simulink library "csc_sim_mtv_simulation_lib"  (R2014b)
settings: Solver=ode45  StartTime=0.0  StopTime=10.0  RelTol=1e-3
undefined symbols (not defined in the file or in its folder): ini_epoch_seconds, sim_time_step_size, swm_num_switches
libraries: util_common_lib x4, util_info_lib x1, telem_conversion_lib x1, csc_egt_egc_thruster_lib x1, csc_enf_environmental_forces_mtv_lib x1, csc_prs_pressure_system_sim_lib x1, csc_pwr_power_system_sim_lib x1, csc_rigid_body_dynamics_lib x1, csc_sensors_mtv_lib x1, csc_thl_thrusters_mtv_lib x1, csc_thm_thermal_system_sim_lib x1, csu_afm_aerodynamics_lib x1
settings Model: Creator=nkulkarni  LastModifiedBy=Mark Wells

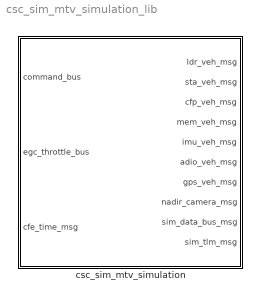
== system csc_sim_mtv_simulation_lib ==
  csc_sim_mtv_simulation : Subsystem  Tag=GSSE; MDL_TICK=THR_SIM_MSG  TreatAsAtomicUnit=on  SystemSampleTime=sim_time_step_size

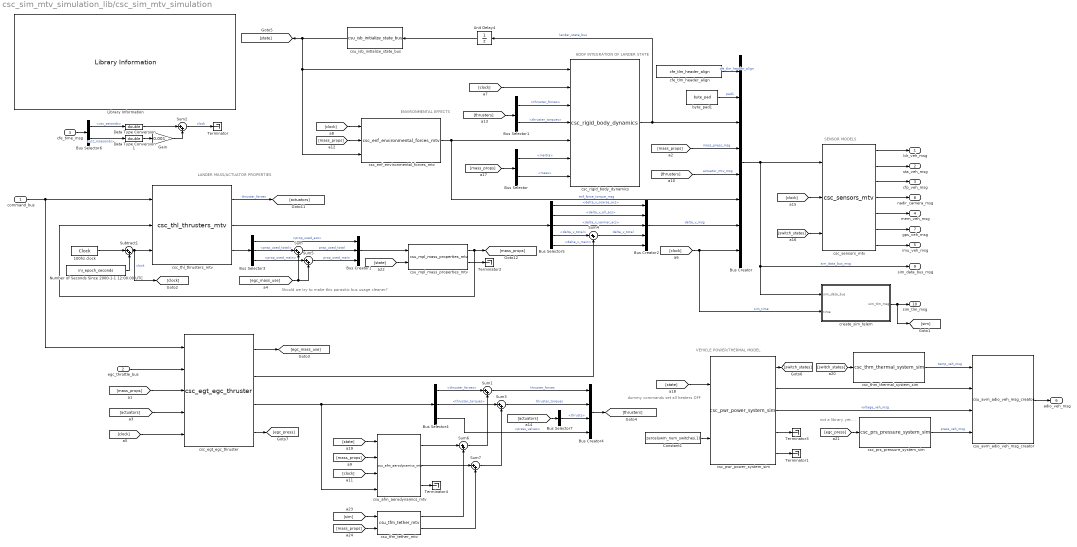
== system csc_sim_mtv_simulation_lib/csc_sim_mtv_simulation ==
  note: Should we try to make this parasitic bus usage cleaner?
  note: SENSOR MODELS
  note: ENVIRONMENTAL EFFECTS
  note: 6DOF INTEGRATION OF LANDER STATE
  note: LANDER MASS/ACTUATOR PROPERTIES
  note: dummy commands set all heaters OFF
  note: VEHICLE POWER/THERMAL MODEL
  note: not a library yet....
  command_bus : Inport
  egc_throttle_bus : Inport  Port=2
  cfe_time_msg : Inport  Port=3  OutDataTypeStr=Bus: cfe_time_msg
  100hz clock : DigitalClock  SampleTime=sim_time_step_size
  Bus Creator : BusCreator  Inputs=8  OutDataTypeStr=Bus: sim_data_mtv_msg  NonVirtualBus=on
  Bus Creator1 : BusCreator  Inputs=3
  Bus Creator2 : BusCreator  Inputs=5
  Bus Creator4 : BusCreator  OutDataTypeStr=Bus: actuator_mtv_msg_t
  Bus Selector : BusSelector  OutputSignals=inertia,mass
  Bus Selector1 : BusSelector  OutputSignals=thruster_forces,thruster_torques
  Bus Selector3 : BusSelector  OutputSignals=prop_used_acs,prop_used_total,prop_used_main
  Bus Selector4 : BusSelector  OutputSignals=thruster_forces,thruster_torques,press_valves
  Bus Selector5 : BusSelector  OutputSignals=delta_v_coarse_acs,delta_v_all_acs,delta_v_vernier_acs,delta_v_total,delta_v_main
  Bus Selector6 : BusSelector  OutputSignals=utc_seconds,utc_mseconds
  Bus Selector7 : BusSelector  OutputSignals=thrusts
  Constant1 : Constant  Value=zeros(swm_num_switches,1)  OutDataTypeStr=double
  Data Type Conversion : DataTypeConversion  OutDataTypeStr=double
  Data Type Conversion1 : DataTypeConversion  OutDataTypeStr=double
  Gain : Gain  Gain=0.001
  Library Information : util_info_lib/Library Information  owner='NONE'
  Number of Seconds Since 2000-1-1 12:00:00 UTC : Constant  Description=|  Value=ini_epoch_seconds
      | Number of Seconds                   
      | July 4, 2014 22:40:00 UTC           
      | Calculate on Web Site:              
      | www.mbari.org/staff/rich/utccalc.htm
  Subtract1 : Sum  Inputs=|++
  Sum{,1..7} (8 alike) : Sum  Inputs=|++
  Terminator{,1..4} (5 alike) : Terminator
  Unit Delay4 : UnitDelay  SampleTime=-1
  byte_pad1 : util_common_lib/byte_pad  n_bytes=4
  cfe_tlm_header_align : util_common_lib/cfe_tlm_header_align
  create_sim_telem : Subsystem
  csc_egt_egc_thruster : csc_egt_egc_thruster_lib/csc_egt_egc_thruster
  csc_enf_environmental_forces_mtv : csc_enf_environmental_forces_mtv_lib/csc_enf_environmental_forces_mtv
  csc_prs_pressure_system_sim : csc_prs_pressure_system_sim_lib/csc_prs_pressure_system_sim
  csc_pwr_power_system_sim : csc_pwr_power_system_sim_lib/csc_pwr_power_system_sim
  csc_rigid_body_dynamics : csc_rigid_body_dynamics_lib/csc_rigid_body_dynamics
  csc_sensors_mtv : csc_sensors_mtv_lib/csc_sensors_mtv
  csc_thl_thrusters_mtv : csc_thl_thrusters_mtv_lib/csc_thl_thrusters_mtv
  csc_thm_thermal_system_sim : csc_thm_thermal_system_sim_lib/csc_thm_thermal_system_sim
  csu_afm_aerodynamics_mtv : csu_afm_aerodynamics_lib/csu_afm_aerodynamics_mtv  SystemSampleTime=-1
  csu_avm_adio_veh_msg_creator : csu_avm_adio_veh_msg_creator_lib/csu_avm_adio_veh_msg_creator
  csu_isb_initialize_state_bus : csu_isb_initialize_state_bus_lib/csu_isb_initialize_state_bus
  csu_mpl_mass_properties_mtv : csu_mpl_mass_properties_mtv_lib/csu_mpl_mass_properties_mtv
  csu_tfm_tether_mtv : csu_tfm_tether_mtv/csu_tfm_tether_mtv
  ldr_veh_msg : Outport
  sta_veh_msg : Outport  Port=2
  cfp_veh_msg : Outport  Port=3
  mem_veh_msg : Outport  Port=4
  imu_veh_msg : Outport  Port=5
  adio_veh_msg : Outport  Port=6
  gps_veh_msg : Outport  Port=7
  nadir_camera_msg : Outport  Port=8
  sim_data_bus_msg : Outport  Port=9
  sim_tlm_msg : Outport  Port=10
  wires:
  Sum7/1 -> Sum3/2
  Sum6/1 -> Sum1/2
  csu_tfm_tether_mtv/2 -> Sum7/2
  csu_afm_aerodynamics_mtv/2 -> Sum7/1
  csu_tfm_tether_mtv/1 -> Sum6/2
  csu_afm_aerodynamics_mtv/1 -> Sum6/1
  [sim] -> csu_tfm_tether_mtv/1
  [mass_props] -> csu_tfm_tether_mtv/2
  Bus Selector4/2 -> Sum3/1  "<thruster_torques>"
  Bus Selector4/1 -> Sum1/1  "<thruster_forces>"
  [state] -> csu_afm_aerodynamics_mtv/1
  [mass_props] -> csu_afm_aerodynamics_mtv/2
  csc_sensors_mtv/7 -> imu_veh_msg/1
  [state] -> csu_mpl_mass_properties_mtv/2
  csc_sensors_mtv/6 -> gps_veh_msg/1
  csu_mpl_mass_properties_mtv/2 -> Terminator2/1
  Bus Selector4/3 -> Bus Creator4/4  "<press_valves>"
  Sum5/1 -> Bus Creator1/3  "prop_used_main"
  [clock] -> csc_egt_egc_thruster/5
  command_bus/1 -> csc_thl_thrusters_mtv/1, csc_egt_egc_thruster/1
  csc_egt_egc_thruster/4 -> [egc_press]
  csc_prs_pressure_system_sim/1 -> csu_avm_adio_veh_msg_creator/4  "press_veh_msg"
  [egc_press] -> csc_prs_pressure_system_sim/1
  csc_pwr_power_system_sim/3 -> csu_avm_adio_veh_msg_creator/3  "voltage_veh_msg"
  csc_pwr_power_system_sim/2 -> csu_avm_adio_veh_msg_creator/2
  csc_thm_thermal_system_sim/1 -> csu_avm_adio_veh_msg_creator/1  "temp_veh_msg"
  csu_avm_adio_veh_msg_creator/1 -> adio_veh_msg/1
  [switch_states] -> csc_thm_thermal_system_sim/1
  Sum2/1 -> Terminator/1  "clock"
  100hz clock/1 -> Subtract1/1
  Number of Seconds Since 2000-1-1 12:00:00 UTC/1 -> Subtract1/2
  csc_sensors_mtv/5 -> mem_veh_msg/1
  [mass_props] -> csc_enf_environmental_forces_mtv/2
  [clock] -> csc_enf_environmental_forces_mtv/1
  csc_thl_thrusters_mtv/1 -> [actuators]  "thruster_forces"
  csc_enf_environmental_forces_mtv/1 -> Bus Creator/6, csc_rigid_body_dynamics/5  "enf_force_torque_msg"
  Bus Selector1/2 -> csc_rigid_body_dynamics/4  "<thruster_torques>"
  Bus Selector1/1 -> csc_rigid_body_dynamics/3  "<thruster_forces>"
  csu_mpl_mass_properties_mtv/1 -> [mass_props], csc_thl_thrusters_mtv/2
  Bus Selector/1 -> csc_rigid_body_dynamics/6  "<inertia>"
  Bus Selector/2 -> csc_rigid_body_dynamics/7  "<mass>"
  [mass_props] -> Bus Creator/4  "mass_props_msg"
  [thrusters] -> Bus Creator/5  "actuator_mtv_msg"
  [thrusters] -> Bus Selector1/1
  [mass_props] -> Bus Selector/1
  csc_rigid_body_dynamics/1 -> Bus Creator/3, Unit Delay4/1  "lander_state_bus"
  Bus Creator/1 -> csc_sensors_mtv/1, sim_data_bus_msg/1, create_sim_telem/1(sim_data_bus)  "sim_data_bus_msg"
  create_sim_telem/1(sim_tlm_msg) -> sim_tlm_msg/1, [sim]
  [clock] -> create_sim_telem/2(time), Bus Creator/8  "sim_time"
  Subtract1/1 -> csc_thl_thrusters_mtv/3, [clock]  "clock"
  byte_pad1/1 -> Bus Creator/2  "pad1"
  csc_thl_thrusters_mtv/3 -> Bus Selector3/1
  csc_egt_egc_thruster/1 -> [egc_mass_use]
  Bus Selector3/2 -> Sum/1  "<prop_used_total>"
  [egc_mass_use] -> Sum/2, Sum5/2
  Sum/1 -> Bus Creator1/2  "prop_used_total"
  Bus Selector3/1 -> Bus Creator1/1  "<prop_used_acs>"
  Bus Selector3/3 -> Sum5/1  "<prop_used_main>"
  Bus Creator1/1 -> csu_mpl_mass_properties_mtv/1
  csc_egt_egc_thruster/2 -> Sum4/2
  Bus Creator2/1 -> Bus Creator/7  "delta_v_msg"
  csc_thl_thrusters_mtv/2 -> Bus Selector5/1
  Bus Selector5/4 -> Sum4/1  "<delta_v_total>"
  Sum4/1 -> Bus Creator2/4  "delta_v_total"
  Bus Selector5/5 -> Bus Creator2/5  "<delta_v_main>"
  Bus Selector5/3 -> Bus Creator2/3  "<delta_v_vernier_acs>"
  Bus Selector5/2 -> Bus Creator2/2  "<delta_v_all_acs>"
  Bus Selector5/1 -> Bus Creator2/1  "<delta_v_coarse_acs>"
  [actuators] -> csc_egt_egc_thruster/4
  [mass_props] -> csc_egt_egc_thruster/3
  egc_throttle_bus/1 -> csc_egt_egc_thruster/2
  cfe_time_msg/1 -> Bus Selector6/1
  Bus Selector6/2 -> Data Type Conversion1/1  "<utc_mseconds>"
  Data Type Conversion/1 -> Sum2/1
  Data Type Conversion1/1 -> Gain/1
  Gain/1 -> Sum2/2
  Bus Selector6/1 -> Data Type Conversion/1  "<utc_seconds>"
  csc_sensors_mtv/1 -> ldr_veh_msg/1
  csc_sensors_mtv/2 -> sta_veh_msg/1
  csc_sensors_mtv/3 -> cfp_veh_msg/1
  csc_sensors_mtv/4 -> nadir_camera_msg/1
  cfe_tlm_header_align/1 -> Bus Creator/1  "cfe_tlm_header_align"
  [clock] -> csc_rigid_body_dynamics/2
  csu_isb_initialize_state_bus/1 -> [state], csc_rigid_body_dynamics/1, csc_enf_environmental_forces_mtv/3
  Unit Delay4/1 -> csu_isb_initialize_state_bus/1
  [clock] -> csc_sensors_mtv/2
  Constant1/1 -> csc_pwr_power_system_sim/2
  [state] -> csc_pwr_power_system_sim/1
  csc_pwr_power_system_sim/1 -> [switch_states]
  csc_pwr_power_system_sim/4 -> Terminator3/1
  csc_pwr_power_system_sim/5 -> Terminator1/1
  [switch_states] -> csc_sensors_mtv/3
  csc_egt_egc_thruster/3 -> csu_afm_aerodynamics_mtv/4, Bus Selector4/1
  Sum1/1 -> Bus Creator4/1  "thruster_forces"
  Bus Creator4/1 -> [thrusters]
  [actuators] -> Bus Selector7/1
  Bus Selector7/1 -> Bus Creator4/3  "<thrusts>"
  Sum3/1 -> Bus Creator4/2  "thruster_torques"
  [clock] -> csu_afm_aerodynamics_mtv/3
  csu_afm_aerodynamics_mtv/3 -> Terminator4/1

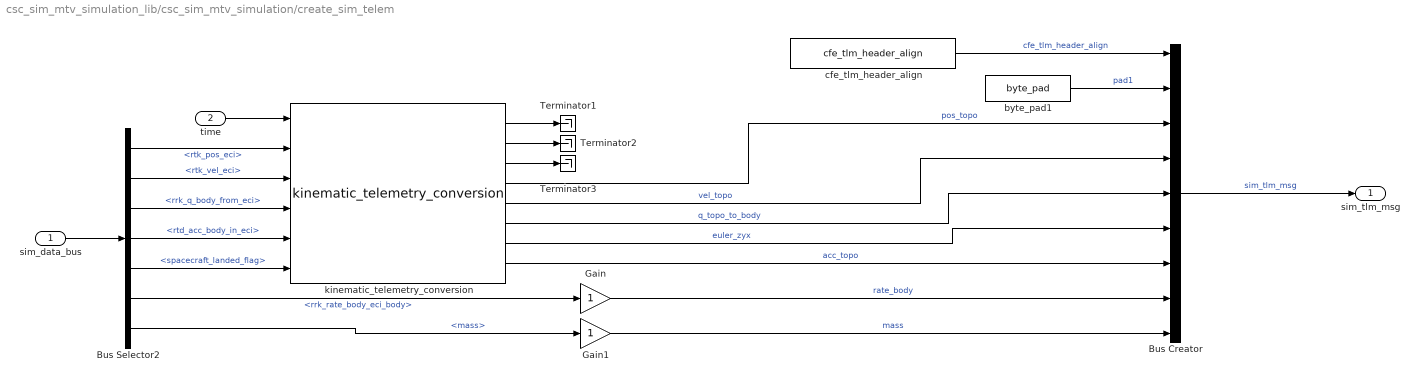
== system csc_sim_mtv_simulation_lib/csc_sim_mtv_simulation/create_sim_telem ==
  sim_data_bus : Inport
  time : Inport  Port=2
  Bus Creator : BusCreator  Inputs=9  OutDataTypeStr=Bus: sim_tlm_msg  NonVirtualBus=on
  Bus Selector2 : BusSelector  OutputSignals=lander_state_bus.rtk_pos_eci,lander_state_bus.rtk_vel_eci,lander_state_bus.rrk_q_body_from_eci,lander_state_bus.rtd_acc_body_in_eci,lander_state_bus.spacecraft_landed_flag,lander_state_bus.rrk_rate_body_eci_body,mass_props_msg.mass
  Gain : Gain
  Gain1 : Gain
  Terminator1 : Terminator
  Terminator2 : Terminator
  Terminator3 : Terminator
  byte_pad1 : util_common_lib/byte_pad  n_bytes=4
  cfe_tlm_header_align : util_common_lib/cfe_tlm_header_align
  kinematic_telemetry_conversion : telem_conversion_lib/kinematic_telemetry_conversion
  sim_tlm_msg : Outport
  wires:
  Bus Selector2/5 -> kinematic_telemetry_conversion/6  "<spacecraft_landed_flag>"
  kinematic_telemetry_conversion/4 -> Bus Creator/3  "pos_topo"
  Gain1/1 -> Bus Creator/9  "mass"
  Bus Selector2/7 -> Gain1/1  "<mass>"
  Gain/1 -> Bus Creator/8  "rate_body"
  Bus Selector2/6 -> Gain/1  "<rrk_rate_body_eci_body>"
  Bus Selector2/4 -> kinematic_telemetry_conversion/5  "<rtd_acc_body_in_eci>"
  Bus Selector2/3 -> kinematic_telemetry_conversion/4  "<rrk_q_body_from_eci>"
  Bus Selector2/2 -> kinematic_telemetry_conversion/3  "<rtk_vel_eci>"
  Bus Selector2/1 -> kinematic_telemetry_conversion/2  "<rtk_pos_eci>"
  time/1 -> kinematic_telemetry_conversion/1
  sim_data_bus/1 -> Bus Selector2/1
  kinematic_telemetry_conversion/5 -> Bus Creator/4  "vel_topo"
  kinematic_telemetry_conversion/6 -> Bus Creator/5  "q_topo_to_body"
  kinematic_telemetry_conversion/7 -> Bus Creator/6  "euler_zyx"
  kinematic_telemetry_conversion/8 -> Bus Creator/7  "acc_topo"
  Bus Creator/1 -> sim_tlm_msg/1  "sim_tlm_msg"
  kinematic_telemetry_conversion/1 -> Terminator1/1
  kinematic_telemetry_conversion/2 -> Terminator2/1
  kinematic_telemetry_conversion/3 -> Terminator3/1
  byte_pad1/1 -> Bus Creator/2  "pad1"
  cfe_tlm_header_align/1 -> Bus Creator/1  "cfe_tlm_header_align"
